simulink model "test_event_sorter"  (R2024a)
settings: Solver=FixedStepDiscrete  StartTime=0.0  StopTime=10  FixedStep=0.1  MaxStep=1  RelTol=1e-3
libraries: dspsrcs4 x1, sldrtlib x1
settings Model: Creator=mfussi  LastModifiedBy=mfussi

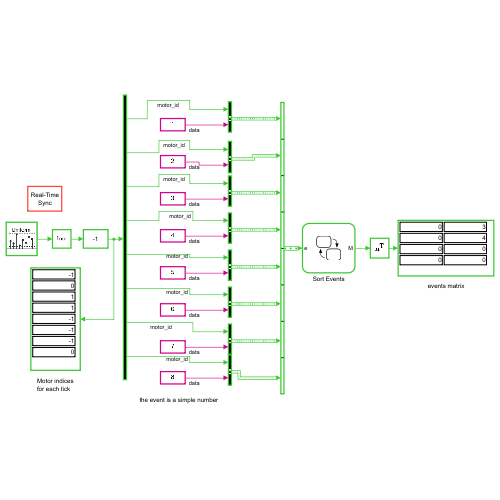
[thumbnail: Simulink's stored preview of the top-level diagram]
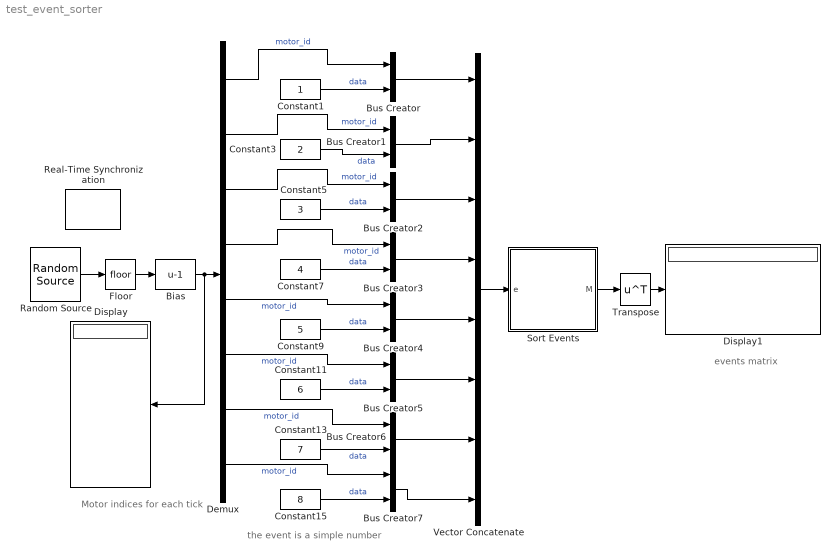
== system test_event_sorter ==
  note: the event is a simple number
  note: events matrix
  note: Motor indices
      | for each tick
  Bias : Bias  Bias=-1  SaturateOnIntegerOverflow=off
  Bus Creator{,1..7} (8 alike) : BusCreator  Inputs=2  OutDataTypeStr=Bus: evt  NonVirtualBus=on
  Constant1 : Constant
  Constant11 : Constant  Value=6
  Constant13 : Constant  Value=7
  Constant15 : Constant  Value=8
  Constant3 : Constant  Value=2
  Constant5 : Constant  Value=3
  Constant7 : Constant  Value=4
  Constant9 : Constant  Value=5
  Demux : Demux  Outputs=8
  Display : Display
  Display1 : Display
  Floor : Rounding
  Random Source : dspsrcs4/Random Source  SrcType=Uniform  MinVal=zeros(1, 8)  MaxVal=ones(1, 8) * 3  MeanVal=0  VarVal=ones(1,8)  RepMode=Not repeatable  rawSeed=1  IsInherit=off  SampTime=1  SampFrame=1  OutComplex=Real  DataType=double  SimulateUsing=Interpreted execution
  Real-Time Synchronization : sldrtlib/Real-Time Synchronization  SampleTime=0.1  MaxMissedTicks=10  ShowMissedTicks=off  YieldWhenWaiting=off
  Sort Events : Stateflow chart  TreatAsAtomicUnit=on
  Transpose : Math  Operator=transpose
  Vector Concatenate : Concatenate  NumInputs=8
  wires:
  Demux/1 -> Bus Creator/1  "motor_id"
  Constant1/1 -> Bus Creator/2  "data"
  Demux/2 -> Bus Creator1/1  "motor_id"
  Constant3/1 -> Bus Creator1/2  "data"
  Constant5/1 -> Bus Creator2/2  "data"
  Demux/3 -> Bus Creator2/1  "motor_id"
  Demux/4 -> Bus Creator3/1  "motor_id"
  Constant7/1 -> Bus Creator3/2  "data"
  Demux/5 -> Bus Creator4/1  "motor_id"
  Constant9/1 -> Bus Creator4/2  "data"
  Demux/6 -> Bus Creator5/1  "motor_id"
  Constant11/1 -> Bus Creator5/2  "data"
  Demux/7 -> Bus Creator6/1  "motor_id"
  Constant13/1 -> Bus Creator6/2  "data"
  Constant15/1 -> Bus Creator7/2  "data"
  Demux/8 -> Bus Creator7/1  "motor_id"
  Random Source/1 -> Floor/1
  Bus Creator7/1 -> Vector Concatenate/8
  Bus Creator/1 -> Vector Concatenate/1
  Bus Creator1/1 -> Vector Concatenate/2
  Bus Creator2/1 -> Vector Concatenate/3
  Bus Creator3/1 -> Vector Concatenate/4
  Bus Creator4/1 -> Vector Concatenate/5
  Bus Creator5/1 -> Vector Concatenate/6
  Bus Creator6/1 -> Vector Concatenate/7
  Vector Concatenate/1 -> Sort Events/1(e)
  Sort Events/1(M) -> Transpose/1
  Transpose/1 -> Display1/1
  Floor/1 -> Bias/1
  Bias/1 -> Display/1, Demux/1

== stateflow chart test_event_sorter/Sort Events ==
  settings: initializeOutput=1
  (default) -> (junction 13) : % Bin Events
  (junction 13) -> (junction 15) : {idx = 0;
      | counter_motor_1 = 0;
      | counter_motor_2 = 0;}
  (junction 15) -> (junction 14) [order 1] : [idx < 2*4]
  (junction 14) -> (junction 60) [order 1] : [e[idx].motor_id == 0 && counter_motor_1 < 4]{
      | M[e[idx].motor_id][counter_motor_1] = e[idx].data;
      | counter_motor_1++;}
  (junction 14) -> (junction 61) [order 2] : [e[idx].motor_id == 1 && counter_motor_2 < 4]{
      | M[e[idx].motor_id][counter_motor_2 ] = e[idx].data;
      | counter_motor_2++;}
  (junction 17) -> (junction 15) : {idx++;}
  (junction 14) -> (junction 17) [order 3]
  (junction 60) -> (junction 61)
  (junction 15) -> (junction 59) [order 2]
  (junction 61) -> (junction 17)
  data: e input Bus: evt size=[2*4]; M output double size=[2, 4]; idx local uint8 size=1; counter_motor_1 local uint8 size=1; counter_motor_2 local uint8 size=1
